simulink model "dynsim_test_urdf_semplice"  (R2020a)
settings: Solver=FixedStepAuto  StartTime=0.0  StopTime=5  FixedStep=0.001  RelTol=1e-3
libraries: robotmaniplib x1
settings Model: Creator=bascetta  LastModifiedBy=alberto
settings OptimizationCC: EnhancedBackFolding=on  PassReuseOutputArgsAs=Individual arguments  ZeroExternalMemoryAtStartup=off  ZeroInternalMemoryAtStartup=off  MaxStackSize=64  OptimizeBlockOrder=speed  DifferentSizesBufferReuse=on  OptimizationCustomize=off  EfficientTunableParamExpr=on
settings DebuggingCC: ParameterTunabilityLossMsg=error
settings HardwareCC: ProdBitPerPointer=32  ProdBitPerSizeT=32  ProdBitPerPtrDiffT=32  ProdLargestAtomicFloat=None  ProdIntDivRoundTo=Undefined  ProdEndianess=Unspecified  ProdWordSize=32  ProdHWDeviceType=Generic->Unspecified (assume 32-bit Generic)
settings RTWCC: SystemTargetFile=ert.tlc  HardwareBoard=Robot Operating System (ROS)  TemplateMakefile=ert_default_tmf  GenerateReport=on  Toolchain=Catkin  IncludeHyperlinkInReport=on  LaunchReport=on  TargetLang=C++  GenerateTraceInfo=on  GenerateTraceReport=on  GenerateTraceReportSl=on  GenerateTraceReportSf=on  GenerateTraceReportEml=on
settings CodeAppCC: ForceParamTrailComments=on  IgnoreCustomStorageClasses=off  OperatorAnnotations=on  SimulinkDataObjDesc=on  SFDataObjDesc=on  InsertBlockDesc=on
settings ERTTargetCC: SupportContinuousTime=on  SupportVariableSizeSignals=on

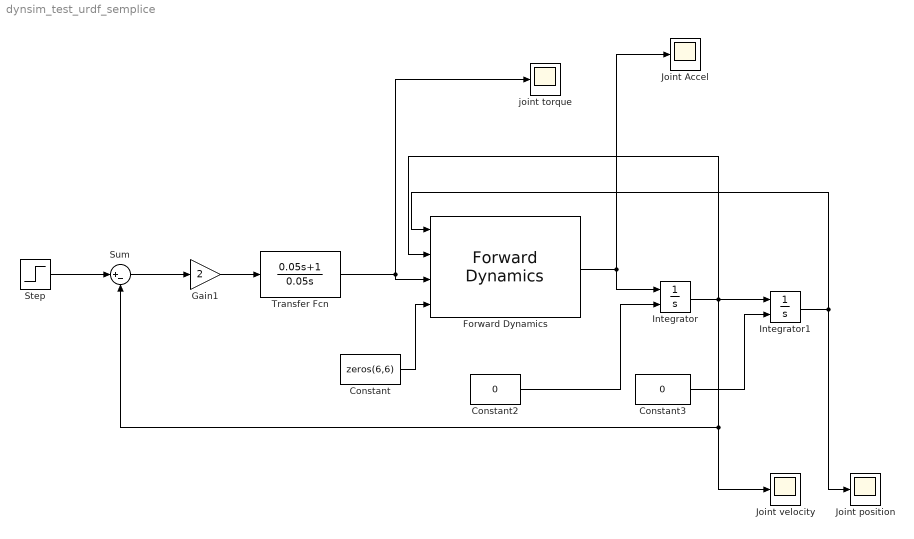
== system dynsim_test_urdf_semplice ==
  Constant : Constant  Value=zeros(6,6)
  Constant2 : Constant  Value=0
  Constant3 : Constant  Value=0
  Forward Dynamics : robotmaniplib/Forward Dynamics  RigidBodyTree=robot_edo_nuove_inerzie  SimulateUsing=Interpreted execution
  Gain1 : Gain  Gain=2
  Integrator : Integrator  InitialConditionSource=external
  Integrator1 : Integrator  InitialConditionSource=external
  Joint Accel : Scope
  Joint position : Scope
  Joint velocity : Scope
  Step : Step  SampleTime=0
  Sum : Sum  Inputs=|+-
  Transfer Fcn : TransferFcn  Numerator=[0.05 1]  Denominator=[0.05 0]
  joint torque : Scope
  wires:
  Constant/1 -> Forward Dynamics/4
  Forward Dynamics/1 -> Integrator/1, Joint Accel/1
  Integrator1/1 -> Forward Dynamics/1, Joint position/1
  Constant2/1 -> Integrator/2
  Constant3/1 -> Integrator1/2
  Integrator/1 -> Sum/2, Joint velocity/1, Forward Dynamics/2, Integrator1/1
  Transfer Fcn/1 -> Forward Dynamics/3, joint torque/1
  Sum/1 -> Gain1/1
  Gain1/1 -> Transfer Fcn/1
  Step/1 -> Sum/1
